simulink model "GANTRY_SYSID"  (R2024b)
settings: Solver=FixedStepAuto  StartTime=0.0  StopTime=inf  FixedStep=1/200  RelTol=1e-3  EnableMultiTasking=on
libraries: mbedblockslib x8
settings Model: ExtModeTrigDuration=10  Creator=patri  LastModifiedBy=Jaylen
settings SolverCC: AutoInsertRateTranBlk=on
settings OptimizationCC: EnhancedBackFolding=on  PassReuseOutputArgsAs=Individual arguments  ZeroExternalMemoryAtStartup=off  ZeroInternalMemoryAtStartup=off  MaxStackSize=64  OptimizeBlockOrder=speed  DifferentSizesBufferReuse=on  OptimizationCustomize=off  EfficientTunableParamExpr=on
settings DebuggingCC: ParameterTunabilityLossMsg=error
settings HardwareCC: ProdBitPerPointer=32  ProdBitPerSizeT=32  ProdBitPerPtrDiffT=32  ProdLargestAtomicInteger=Long  ProdLargestAtomicFloat=Double  ProdWordSize=32  ProdLongLongMode=on  ProdHWDeviceType=ARM Compatible->ARM Cortex-M
settings SFSimCC: MATLABDynamicMemAlloc=off
settings RTWCC: Description=Embedded Coder  SystemTargetFile=ert.tlc  HardwareBoard=STM32 Nucleo F767ZI  TemplateMakefile=ert_default_tmf  Toolchain=GNU Tools for ARM Embedded Processors
settings CodeAppCC: ForceParamTrailComments=on  IgnoreCustomStorageClasses=off  OperatorAnnotations=on  SimulinkDataObjDesc=on  SFDataObjDesc=on  InsertBlockDesc=on
settings ERTTargetCC: ExtModeTransport=3  ExtModeStaticAlloc=on  ExtModeStaticAllocSize=10000  ExtModeMexFile=ext_xcp  ExtModeIntrfLevel=Level2 - Open  InlinedParameterPlacement=Hierarchical

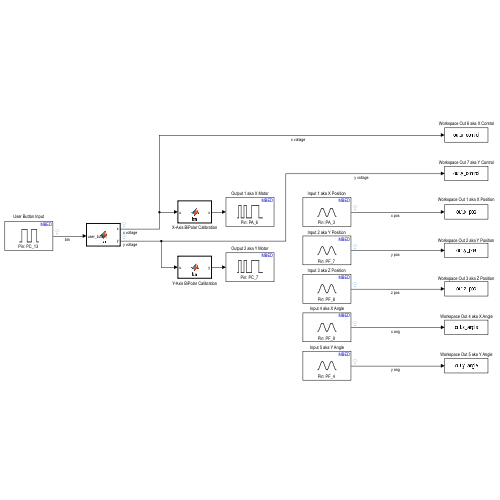
[thumbnail: Simulink's stored preview of the top-level diagram]
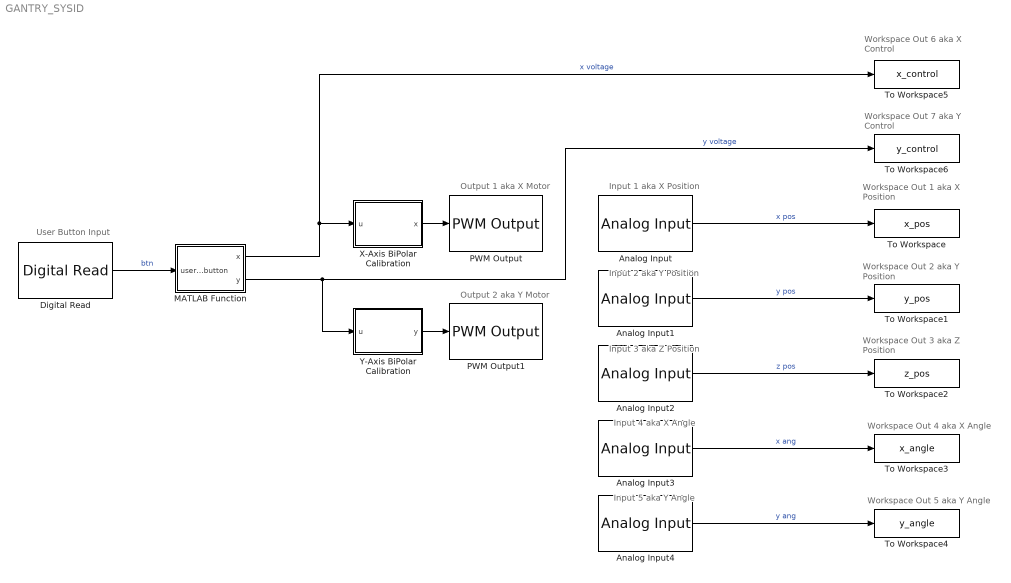
== system GANTRY_SYSID ==
  note: Input 1 aka X Position
  note: User Button Input
  note: Input 2 aka Y Position
  note: Input 3 aka Z Position
  note: Workspace Out 1 aka X Position
  note: Input 5 aka Y Angle
  note: Input 4 aka X Angle
  note: Workspace Out 6 aka X Control
  note: Workspace Out 7 aka Y Control
  note: Workspace Out 5 aka Y Angle
  note: Workspace Out 3 aka Z Position
  note: Workspace Out 4 aka X Angle
  note: Workspace Out 2 aka Y Position
  note: Output 1 aka X Motor
  note: Output 2 aka Y Motor
  Analog Input : mbedblockslib/Analog Input  Pin=PA_3  ReadResultsOnly=off  ConversionTriggerSource=Software  ExternalTriggerType=uint32( 0 )  OutputDataType=double  EnableConversionCompleteNotify=off  EnableOuputStatus=off  SampleTime=-1
      settings: LibrarySourceBlock=stmnucleorootlib/Common/Analog Input
  Analog Input1 : mbedblockslib/Analog Input  Pin=PF_7  ReadResultsOnly=off  ConversionTriggerSource=Software  ExternalTriggerType=uint32( 0 )  OutputDataType=double  EnableConversionCompleteNotify=off  EnableOuputStatus=off  SampleTime=-1
      settings: LibrarySourceBlock=stmnucleorootlib/Common/Analog Input
  Analog Input2 : mbedblockslib/Analog Input  Pin=PF_8  ReadResultsOnly=off  ConversionTriggerSource=Software  ExternalTriggerType=uint32( 0 )  OutputDataType=double  EnableConversionCompleteNotify=off  EnableOuputStatus=off  SampleTime=-1
      settings: LibrarySourceBlock=stmnucleorootlib/Common/Analog Input
  Analog Input3 : mbedblockslib/Analog Input  Pin=PF_9  ReadResultsOnly=off  ConversionTriggerSource=Software  ExternalTriggerType=uint32( 0 )  OutputDataType=double  EnableConversionCompleteNotify=off  EnableOuputStatus=off  SampleTime=-1
      settings: LibrarySourceBlock=stmnucleorootlib/Common/Analog Input
  Analog Input4 : mbedblockslib/Analog Input  Pin=PF_4  ReadResultsOnly=off  ConversionTriggerSource=Software  ExternalTriggerType=uint32( 0 )  OutputDataType=double  EnableConversionCompleteNotify=off  EnableOuputStatus=off  SampleTime=-1
      settings: LibrarySourceBlock=stmnucleorootlib/Common/Analog Input
  Digital Read : mbedblockslib/Digital Read  Pin=PC_13  Direction=input  SampleTime=-1
      settings: LibrarySourceBlock=stmnucleorootlib/Common/Digital Read
  MATLAB Function : MATLAB Function  TreatAsAtomicUnit=on
  PWM Output : mbedblockslib/PWM Output  Pin=PA_6  EnableInputFrequency=off  InitialFrequency=10000  InitialDutyCycle=57.6  NotificationType=None
      settings: LibrarySourceBlock=stmnucleorootlib/Common/PWM Output
  PWM Output1 : mbedblockslib/PWM Output  Pin=PC_7  EnableInputFrequency=off  InitialFrequency=10000  InitialDutyCycle=57.6  NotificationType=None
      settings: LibrarySourceBlock=stmnucleorootlib/Common/PWM Output
  To Workspace : ToWorkspace  VariableName=x_pos  SaveFormat=Timeseries  SampleTime=-1
  To Workspace1 : ToWorkspace  VariableName=y_pos  SaveFormat=Timeseries  SampleTime=-1
  To Workspace2 : ToWorkspace  VariableName=z_pos  SaveFormat=Timeseries  SampleTime=-1
  To Workspace3 : ToWorkspace  VariableName=x_angle  SaveFormat=Timeseries  SampleTime=-1
  To Workspace4 : ToWorkspace  VariableName=y_angle  SaveFormat=Timeseries  SampleTime=-1
  To Workspace5 : ToWorkspace  VariableName=x_control  SaveFormat=Timeseries  SampleTime=-1
  To Workspace6 : ToWorkspace  VariableName=y_control  SaveFormat=Timeseries  SampleTime=-1
  X-Axis BiPolar Calibration : MATLAB Function  TreatAsAtomicUnit=on
  Y-Axis BiPolar Calibration : MATLAB Function  TreatAsAtomicUnit=on
  wires:
  Analog Input4/1 -> To Workspace4/1  "y ang"
  Analog Input2/1 -> To Workspace2/1  "z pos"
  Digital Read/1 -> MATLAB Function/1(user_button)  "btn"
  Analog Input/1 -> To Workspace/1  "x pos"
  Analog Input1/1 -> To Workspace1/1  "y pos"
  Analog Input3/1 -> To Workspace3/1  "x ang"
  X-Axis BiPolar Calibration/1(x) -> PWM Output/1
  Y-Axis BiPolar Calibration/1(y) -> PWM Output1/1
  MATLAB Function/1(x) -> To Workspace5/1, X-Axis BiPolar Calibration/1(u)  "x voltage"
  MATLAB Function/2(y) -> Y-Axis BiPolar Calibration/1(u), To Workspace6/1  "y voltage"

== matlab function GANTRY_SYSID/MATLAB Function ==
  data: x output; user_button input; y output
function [x, y] = fcn(user_button)
    % This function generates values for x and y based on the user input.
    % The output x and y depend on a sequence determined by the state variable m and user_button.
    
    % Declare persistent variables that maintain their values between function calls.
    persistent i m button_pressed
    
    % Initialize persistent variables if they are empty.
    if isempty(m)
        m = 0; % m tracks the sequence stage.
        i = 0; % i is used as a time counter.
        button_pressed = 0; % Indicates whether the button was pressed.
    end

    % Sampling frequency (200 Hz)
    Fs = 200;

    % Check if the user has pressed the button (user_button == 1).
    if user_button == 1
        button_pressed = 1; % Set the button pressed flag to 1.
    end

    % Initialize x and y to 0.
    x = 0;
    y = 0;

    % Proceed only if the button has been pressed.
    if button_pressed == 1
        % Sequence control based on the value of m.
        if m == 0
            % Stage 0: x goes from 0 to 10.
            if i < 1 * Fs
                x = 0; % Keep x at 0 for the first second.
            elseif i < 8 * Fs
                x = 10; % Set x to 10 for the next 7 seconds.
            else
                x = 0; % Reset x to 0.
                m = 1; % Move to the next stage.
                i = 0; % Reset the counter.
                button_pressed = 0; % Reset button pressed status.
            end
        elseif m == 1
            % Stage 1: x goes from 0 to -10.
            if i < 1 * Fs
                x = 0; % Keep x at 0 for the first second.
            elseif i < 8 * Fs
                x = -10; % Set x to -10 for the next 7 seconds.
            else
                x = 0; % Reset x to 0.
                m = 2; % Move to the next stage.
                i = 0; % Reset the counter.
                button_pressed = 0; % Reset button pressed status.
            end
        elseif m == 2
            % Stage 2: y goes from 0 to 10.
            if i < 1 * Fs
                y = 0; % Keep y at 0 for the first second.
            elseif i < 8 * Fs
                y = 10; % Set y to 10 for the next 7 seconds.
            else
                y = 0; % Reset y to 0.
                m = 3; % Move to the next stage.
                i = 0; % Reset the counter.
                button_pressed = 0; % Reset button pressed status.
            end
        elseif m == 3
            % Stage 3: y goes from 0 to -10.
            if i < 1 * Fs
                y = 0; % Keep y at 0 for the first second.
            elseif i < 8 * Fs
                y = -10; % Set y to -10 for the next 7 seconds.
            else
                y = 0; % Reset y to 0.
                m = 4; % Move to the next stage.
                i = 0; % Reset the counter.
                button_pressed = 0; % Reset button pressed status.
            end
        else
            % If m is not 0, 1, 2, or 3, do nothing.
            x = 0;
            y = 0;
        end

        % Increment the counter at each function call.
        i = i + 1;
    end
end

== matlab function GANTRY_SYSID/Y-Axis BiPolar Calibration ==
  data: u input; y output
function y = fcn(u)

% Calibration data for y axis output y = p1*u + p2
y = 3.41*u + 59.49;

== matlab function GANTRY_SYSID/X-Axis BiPolar Calibration ==
  data: u input; x output
function x = fcn(u)

% Calibration data for x axis output x = p1*u + p2
x = 2.758*u + 63.834;
